simulink model "ZFE"  (R2022b)
settings: Solver=VariableStepAuto  StartTime=0.0  StopTime=10.0  RelTol=1e-3
undefined symbols (not defined in the file): c, d, L, M, Ns, r, Ts, w
libraries: commfilt2 x3, commsink2 x2, commchan3 x1, dsparch4 x1, commrandsrc3 x1, commutil2 x1
settings Model: Creator=metal  LastModifiedBy=metal

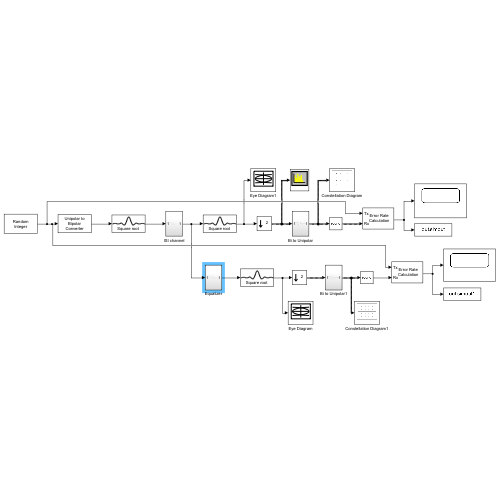
[thumbnail: Simulink's stored preview of the top-level diagram]
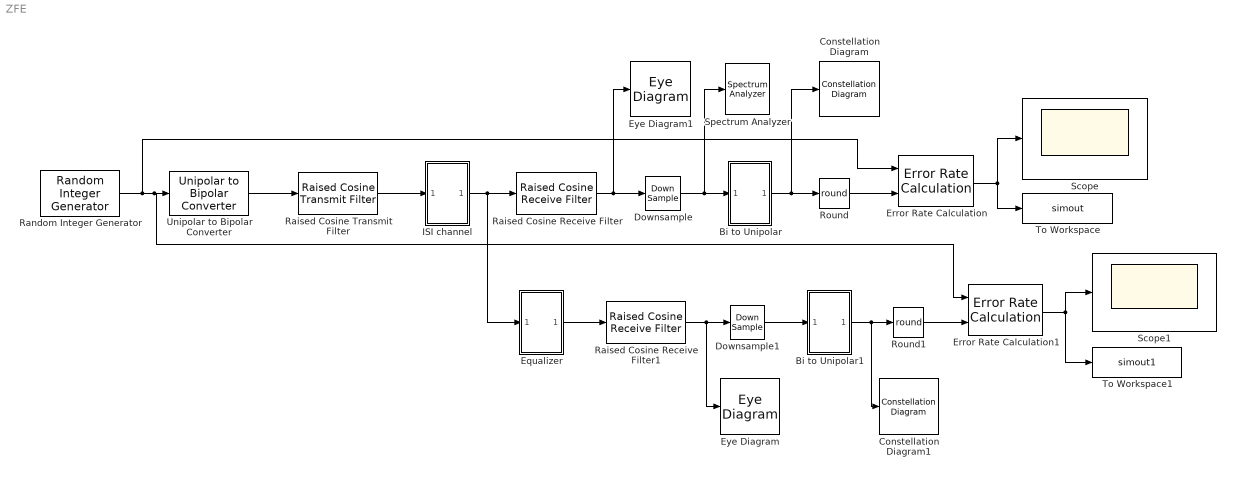
== system ZFE ==
  Bi to Unipolar : Subsystem
  Bi to Unipolar1 : Subsystem
  Constellation Diagram : ConstellationDiagram  WindowPosition=[382.000000,84.000000,600.000000,600.000000,]  ScopeFrameLocation=window  SymbolsToDisplaySource=Property  SymbolsToDisplay=1000  ReferenceConstellation=[0 1 2 3]  XLimits=[-1.46,1.46]  YLimits=[-1.38,1.38]
  Constellation Diagram1 : ConstellationDiagram  WindowPosition=[382.000000,84.000000,600.000000,600.000000,]  ScopeFrameLocation=window  SymbolsToDisplaySource=Property  SymbolsToDisplay=1000  ReferenceConstellation=[0 1 2 3]  XLimits=[-1.3,1.31]  YLimits=[-1.25,1.21]
  Downsample : DownSample  AllowArbitraryFixedInput=on
  Downsample1 : DownSample  AllowArbitraryFixedInput=on
  Equalizer : Subsystem
  Error Rate Calculation : commsink2/Error Rate Calculation  N=L+2  st_delay=0  cp_mode=Entire frame  subframe=[]  PMode=Port  WsName=ErrorVec  RsMode2=off  stop=off  numErr=100  maxBits=1e6
  Error Rate Calculation1 : commsink2/Error Rate Calculation  N=L+2+d  st_delay=0  cp_mode=Entire frame  subframe=[]  PMode=Port  WsName=ErrorVec  RsMode2=off  stop=off  numErr=100  maxBits=1e6
  Eye Diagram : EyeDiagram
  Eye Diagram1 : EyeDiagram
  ISI channel : Subsystem
  Raised Cosine Receive Filter : commfilt2/Raised Cosine Receive Filter  filtType=Square root  R=r  filtSpan=4  N=Ns  downFactor=1  downOffset=0  filterGain=1  InputProcessing=Columns as channels (frame based)  RateOptions=Enforce single-rate processing  framing=Mute  checkCoeff=off  variableName=rcRxFilt  currentFiltSpan=10  D=5  inputOffset=0  sampMode=Mute  saveAsFlag=0  rateMode=Downsampling  checkGain=Normalized  launchFVT=on  roundingMode=Floor  overflowMode=off  coeffDataTypeStr=Inherit: Same word length as input  coeffMin=[]  coeffMax=[]  coeffLastDataTypeStr=Inherit: Same word length as input  accumDataTypeStr=Inherit: Same as product output  accumLastDataTypeStr=Inherit: Same as product output  outputDataTypeStr=Inherit: Same as accumulator  outputMin=[]  outputMax=[]  outputLastDataTypeStr=Inherit: Same as accumulator
  Raised Cosine Receive Filter1 : commfilt2/Raised Cosine Receive Filter  filtType=Square root  R=r  filtSpan=4  N=Ns  downFactor=1  downOffset=0  filterGain=1  InputProcessing=Columns as channels (frame based)  RateOptions=Enforce single-rate processing  framing=Mute  checkCoeff=off  variableName=rcRxFilt1  currentFiltSpan=10  D=5  inputOffset=0  sampMode=Mute  saveAsFlag=0  rateMode=Downsampling  checkGain=Normalized  launchFVT=on  roundingMode=Floor  overflowMode=off  coeffDataTypeStr=Inherit: Same word length as input  coeffMin=[]  coeffMax=[]  coeffLastDataTypeStr=Inherit: Same word length as input  accumDataTypeStr=Inherit: Same as product output  accumLastDataTypeStr=Inherit: Same as product output  outputDataTypeStr=Inherit: Same as accumulator  outputMin=[]  outputMax=[]  outputLastDataTypeStr=Inherit: Same as accumulator
  Raised Cosine Transmit Filter : commfilt2/Raised Cosine Transmit Filter  filtType=Square root  R=r  filtSpan=4  N=Ns  filterGain=1  InputProcessing=Columns as channels (frame based)  RateOptions=Enforce single-rate processing  framing=Mute  checkCoeff=off  variableName=rcTxFilt  checkGain=Normalized  sampMode=Mute  saveAsFlag=0  currentFiltSpan=10  D=(10)/2  launchFVT=on  roundingMode=Floor  overflowMode=off  coeffDataTypeStr=Inherit: Same word length as input  coeffMin=[]  coeffMax=[]  coeffLastDataTypeStr=Inherit: Same word length as input  outputDataTypeStr=Inherit: Same as accumulator  outputMin=[]  outputMax=[]  outputLastDataTypeStr=Inherit: Same as accumulator
  Random Integer Generator : commrandsrc3/Random Integer Generator  SetSize=M  SeedSource=Auto  Seed=0  SampleTime=Ts  SamplesPerFrame=1  OutputDataType=double  SimulateUsing=Interpreted execution
  Round : Rounding  Operator=round
  Round1 : Rounding  Operator=round
  Scope : Scope
  Scope1 : Scope
  Spectrum Analyzer : SpectrumAnalyzer
  To Workspace : ToWorkspace  VariableName=simout  SaveFormat=Timeseries  SampleTime=-1
  To Workspace1 : ToWorkspace  VariableName=simout1  SaveFormat=Timeseries  SampleTime=-1
  Unipolar to Bipolar Converter : commutil2/Unipolar to Bipolar Converter  M=M  polarity=Positive  dataType=Same as input
  wires:
  Random Integer Generator/1 -> Unipolar to Bipolar Converter/1, Error Rate Calculation1/1, Error Rate Calculation/1
  Unipolar to Bipolar Converter/1 -> Raised Cosine Transmit Filter/1
  Error Rate Calculation/1 -> Scope/1, To Workspace/1
  Error Rate Calculation1/1 -> To Workspace1/1, Scope1/1
  Raised Cosine Transmit Filter/1 -> ISI channel/1(In1)
  ISI channel/1(Out1) -> Equalizer/1(In1), Raised Cosine Receive Filter/1
  Raised Cosine Receive Filter/1 -> Downsample/1, Eye Diagram1/1
  Downsample/1 -> Spectrum Analyzer/1, Bi to Unipolar/1(In1)
  Bi to Unipolar/1(Out1) -> Constellation Diagram/1, Round/1
  Round/1 -> Error Rate Calculation/2
  Equalizer/1(Out1) -> Raised Cosine Receive Filter1/1
  Raised Cosine Receive Filter1/1 -> Eye Diagram/1, Downsample1/1
  Downsample1/1 -> Bi to Unipolar1/1(In1)
  Bi to Unipolar1/1(Out1) -> Constellation Diagram1/1, Round1/1
  Round1/1 -> Error Rate Calculation1/2

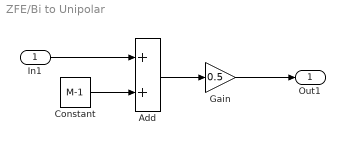
== system ZFE/Bi to Unipolar ==
  In1 : Inport
  Add : Sum
  Constant : Constant  Value=M-1
  Gain : Gain  Gain=0.5
  Out1 : Outport
  wires:
  Gain/1 -> Out1/1
  Add/1 -> Gain/1
  In1/1 -> Add/1
  Constant/1 -> Add/2

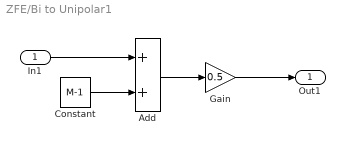
== system ZFE/Bi to Unipolar1 ==
  In1 : Inport
  Add : Sum
  Constant : Constant  Value=M-1
  Gain : Gain  Gain=0.5
  Out1 : Outport
  wires:
  Gain/1 -> Out1/1
  Add/1 -> Gain/1
  In1/1 -> Add/1
  Constant/1 -> Add/2

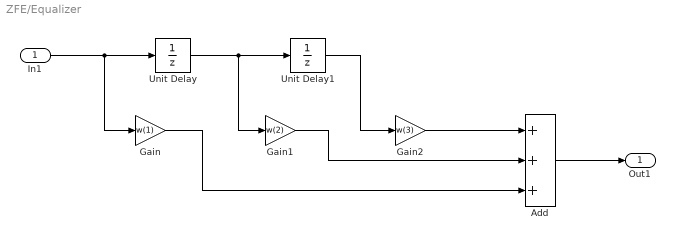
== system ZFE/Equalizer ==
  In1 : Inport
  Add : Sum  Inputs=+++
  Gain : Gain  Gain=w(1)
  Gain1 : Gain  Gain=w(2)
  Gain2 : Gain  Gain=w(3)
  Unit Delay : UnitDelay  SampleTime=Ts  HasFrameUpgradeWarning=on
  Unit Delay1 : UnitDelay  SampleTime=Ts  HasFrameUpgradeWarning=on
  Out1 : Outport
  wires:
  Gain/1 -> Add/3
  Gain2/1 -> Add/1
  Add/1 -> Out1/1
  Unit Delay/1 -> Gain1/1, Unit Delay1/1
  In1/1 -> Gain/1, Unit Delay/1
  Unit Delay1/1 -> Gain2/1
  Gain1/1 -> Add/2

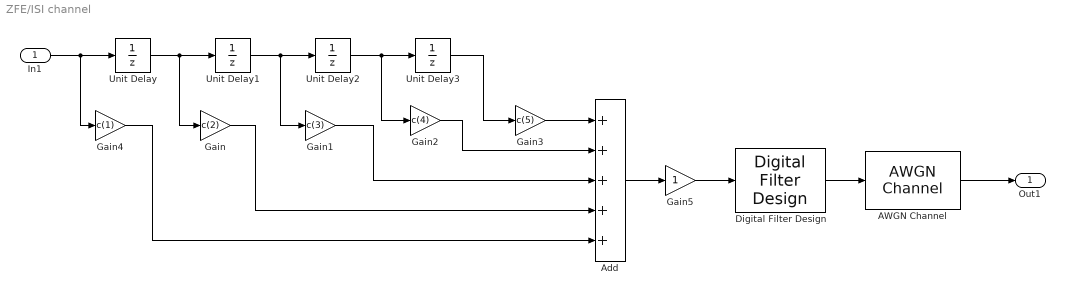
== system ZFE/ISI channel ==
  In1 : Inport
  AWGN Channel : commchan3/AWGN Channel  InputProcessing=Columns as channels (frame based)  seed=21  noiseMode="Signal to noise ratio  (Eb/No)"  EbNodB=EbN0dB  EsNodB=10  SNRdB=10  bitsPerSym=b  Ps=1  Tsym=Ts  variance=1
  Add : Sum  Inputs=+++++
  Digital Filter Design : dsparch4/Digital Filter Design  mwdsp_browser_bugfix_var=off
  Gain : Gain  Gain=c(2)
  Gain1 : Gain  Gain=c(3)
  Gain2 : Gain  Gain=c(4)
  Gain3 : Gain  Gain=c(5)
  Gain4 : Gain  Gain=c(1)
  Gain5 : Gain
  Unit Delay{,1..3} (4 alike) : UnitDelay  SampleTime=Ts  HasFrameUpgradeWarning=on
  Out1 : Outport
  wires:
  Gain1/1 -> Add/3
  AWGN Channel/1 -> Out1/1
  Digital Filter Design/1 -> AWGN Channel/1
  Gain/1 -> Add/4
  Gain3/1 -> Add/1
  Gain4/1 -> Add/5
  Gain2/1 -> Add/2
  Unit Delay2/1 -> Gain2/1, Unit Delay3/1
  Unit Delay1/1 -> Gain1/1, Unit Delay2/1
  Unit Delay3/1 -> Gain3/1
  In1/1 -> Gain4/1, Unit Delay/1
  Gain5/1 -> Digital Filter Design/1
  Unit Delay/1 -> Gain/1, Unit Delay1/1
  Add/1 -> Gain5/1
